simulink model "ex1_fuzzy"  (R2018a)
settings: Solver=ode5  StartTime=0.0  StopTime=20  FixedStep=0.01  RelTol=1e-3
undefined symbols (not defined in the file): sigbuilder_block
libraries: fuzblock x1
settings Model: Creator=DELL  LastModifiedBy=DELL

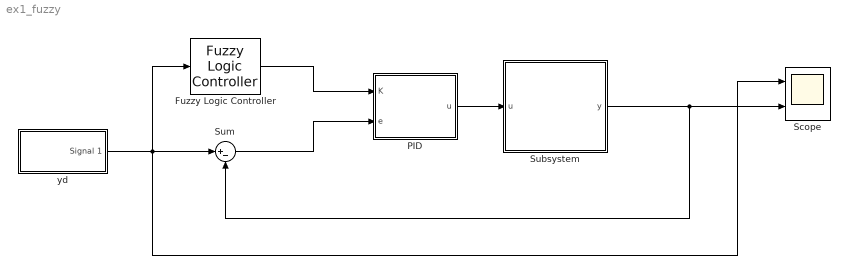
== system ex1_fuzzy ==
  Fuzzy Logic Controller : fuzblock/Fuzzy Logic  Controller  FIS='fuzzy1.fis'  OutputSampleNumber=101  DataType=double  FuzzifiedInputs=off  RuleFiringStrengths=off  RuleOutputs=off  AggregatedOutputs=off  SimulateUsing=Interpreted execution  OutOfRangeInputValueMessage=warning  NoRuleFiredMessage=warning  EmptyOutputFuzzySetMessage=warning
  PID : Subsystem
  Scope : Scope  NumInputPorts=2
  Subsystem : Subsystem  mask{m=1, l=0.6, b=0.1, g=9.81}
      mask prompts: m "khoi luong con lac"; l "chieu dai con lac"; b "he so ma sat"; g "gia toc"
  Sum : Sum  Inputs=|+-
  "yd " : Subsystem  Tag=STV Subsys  LoadFcn=sigbuilder_block('load');  StartFcn=sigbuilder_block('start');  StopFcn=sigbuilder_block('stop');  ClipboardFcn=sigbuilder_block('clipboard');  mask(Sigbuilder block){tuvar=[0:10]}
      mask help: Simulink:masks:SigbuilderBlock_MD
      mask init:
      | if ~strcmp(get_param(bdroot(gcbh),'SimulationStatus'),'stopped') tuvar = sigbuilder_block('maskInit'); end
      settings: CopyFcn=sigbuilder_block('copy');  DeleteFcn=sigbuilder_block('delete');  ModelCloseFcn=sigbuilder_block('modelClose');  PreSaveFcn=sigbuilder_block('preSave');  PauseFcn=sigbuilder_block('pause');  ContinueFcn=sigbuilder_block('continue');  NameChangeFcn=sigbuilder_block('namechange');  OpenFcn=sigbuilder_block('open',[437.6 199.2 550.4 400 ]);  CloseFcn=sigbuilder_block('close');
      mask Display: plot(0, 0, 100, 100,[2, 2, 32, 32, 2], [68, 8, 8, 68, 68],[32, 2], [38, 38], [32, 19, 2],[53, 60, 44], [32, 17, 17, 2],[16, 16, 31, 31]);txt = getActiveGroup(gcbh);text(2, 100, txt,'verticalAlignment', 'top');
  wires:
  PID/1(u) -> Subsystem/1(u)
  Sum/1 -> PID/2(e)
  "yd "/1(Signal 1) -> Sum/1, Fuzzy Logic Controller/1, Scope/1
  Fuzzy Logic Controller/1 -> PID/1(K)
  Subsystem/1(y) -> Scope/2, Sum/2

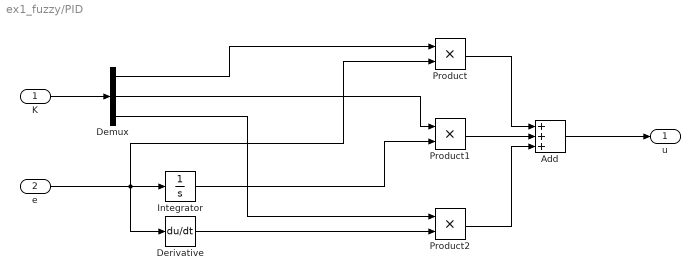
== system ex1_fuzzy/PID ==
  K : Inport
  e : Inport  Port=2
  Add : Sum  Inputs=+++
  Demux : Demux  Outputs=3
  Derivative : Derivative
  Integrator : Integrator
  Product : Product
  Product1 : Product
  Product2 : Product
  u : Outport
  wires:
  K/1 -> Demux/1
  Demux/1 -> Product/1
  e/1 -> Product/2, Integrator/1, Derivative/1
  Integrator/1 -> Product1/2
  Demux/2 -> Product1/1
  Demux/3 -> Product2/1
  Derivative/1 -> Product2/2
  Product/1 -> Add/1
  Product1/1 -> Add/2
  Product2/1 -> Add/3
  Add/1 -> u/1

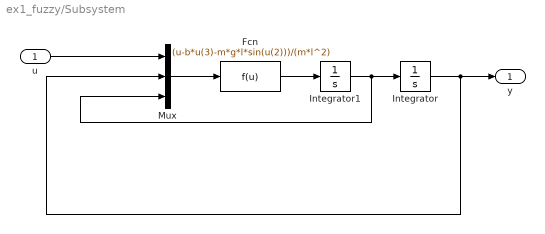
== system ex1_fuzzy/Subsystem ==
  u : Inport
  Fcn : Fcn  Expr=(u-b*u(3)-m*g*l*sin(u(2)))/(m*l^2)
  Integrator : Integrator
  Integrator1 : Integrator
  Mux : Mux  Inputs=3
  y : Outport
  wires:
  Integrator/1 -> Mux/2, y/1
  Fcn/1 -> Integrator1/1
  Mux/1 -> Fcn/1
  u/1 -> Mux/1
  Integrator1/1 -> Mux/3, Integrator/1

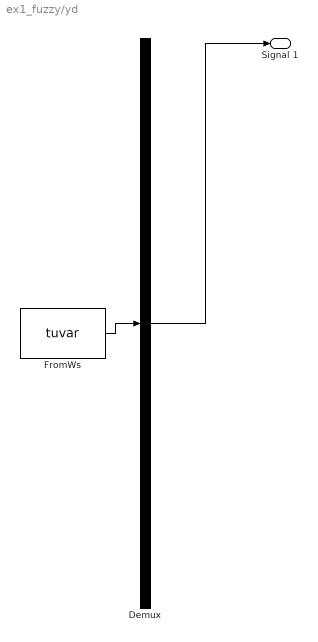
== system ex1_fuzzy/yd  ==
  Demux : Demux  Tag=STV Demux  Outputs=1
  FromWs : FromWorkspace  Tag=STV FromWs  VariableName=tuvar  SampleTime=0
      SigBuilderData=|
      | common.afterFinalStr = 'Extrapolate'
      | common.sampleTime = 0
      | dataSet.timeRange = [0 20]
      | dataSet.name = 'Group 1'
      | sbobj.Groups.Name = 'Group 1'
      | sbobj.Groups.Signals.Name = 'Signal 1'
      | sbobj.Groups.Signals.XData = [0 3.02 3.02 6 6 9.95 9.95 13.95 13.95 20]
      | sbobj.Groups.Signals.YData = [2.3 2.3 1 1 0 0 1.81 1.81 1.23 1.23]
      | sbobj.Groups.TimeRange = [0 20]
  Signal 1 : Outport  Tag=STV Outport
  wires:
  Demux/1 -> Signal 1/1
  FromWs/1 -> Demux/1
